simulink model "raspi_multicore_MPCtest_estDis"  (R2021b)
settings: Solver=FixedStepAuto  StartTime=0.0  StopTime=600  FixedStep=0.006  RelTol=1e-3  EnableMultiTasking=on
InitFcn:
  | %hardwareSetup;
values from neighbouring files (symbols this model uses):
  T_gait = 0.6    [MPCGen_OffsetFree.m]    (also in MPCGen_OffsetFree_UD.m = 0.65; MPCGen_OffsetFree_estDis.m; MPCcontrollerGen_OffsetFree.m = 0.7; MPCcontrollerGen_OffsetFree_UD.m = 0.65)
  Ts = 0.025    [MPCGen_OffsetFree.m]    (also in MPCGen_OffsetFree_UD.m = 0.02; MPCGen_OffsetFree_estDis.m = 0.03; MPCcontrollerGen_OffsetFree.m; MPCcontrollerGen_OffsetFree_UD.m = 0.02)
  Ts_DynSim = 0.005    [MPCGen_OffsetFree.m]    (also in MPCGen_OffsetFree_UD.m; MPCGen_OffsetFree_estDis.m = 0.006; MPCcontrollerGen_OffsetFree.m; MPCcontrollerGen_OffsetFree_UD.m)
libraries: PuppyLibrary x5, mpclib x1, slctrlblks x1
(part 2 of 2)

== matlab function raspi_multicore_MPCtest_estDis/MATLAB Function3 ==
  data: Xnow input; pCoM output; vCoM output; RPY output; Omega output
function [pCoM,vCoM,RPY,Omega] = fcn(Xnow)
pCoM=reshape(Xnow(1:3),3,1);
vCoM=reshape(Xnow(7:9),3,1);
RPY=reshape(Xnow(4:6),3,1);
Omega=reshape(Xnow(10:12),3,1);

== matlab function raspi_multicore_MPCtest_estDis/slopeGen1 ==
  data: slope input; sura output; startX input
function sura = fcn(slope,startX)
slope=slope/180*pi;
surP1=[startX;1;0];
surP2=[startX;-1;0];
surP3=[startX+1;0;tan(slope)];
W=[1,surP1(1:2)';
    1,surP2(1:2)';
    1,surP3(1:2)'];

sura=(W'*W)\W'*[surP1(3);surP2(3);surP3(3);];

== matlab function raspi_multicore_MPCtest_estDis/terrainSimulator1 ==
  data: surP1 input; touchInd output; surP2 input; xBP input; pendAll input; phi input; zSur output
function [touchInd,zSur] = fcn(surP1,surP2,xBP,pendAll,phi)
touchInd=zeros(4,1);
zSur=zeros(4,1);
LegState=[1;0;0;1];
s=phi/pi;
if phi>pi
    LegState=[0;1;1;0];
    s=s-1;
end
for i=1:1:4
    if LegState(i)<0.5 && s>0.2
        if pendAll(1,i)<xBP
            zSur(i)=[1;pendAll(1:2,i)]'*surP1;
        else
            zSur(i)=[1;pendAll(1:2,i)]'*surP2;
        end
        if pendAll(3,i)-zSur(i)<=0.001
            touchInd(i)=1;
        end
    end
end
end

== matlab function raspi_multicore_MPCtest_estDis/MATLAB Function4 ==
  data: SP input; zSur output size=[4,1]; SPLeg input; phi input; touchInd output size=[4,1]; OscStop input; LegState output size=[4,1]
function [zSur,touchInd,LegState] = fcn(SP,SPLeg,phi,OscStop)
zSur=reshape(SP(3,:),4,1);
LegState=[1;0;0;1];
touchInd=SPLeg;
s=phi/pi;
if phi>pi
    s=s-1;
    LegState=[0;1;1;0];
end
if abs(OscStop-1)<0.1
    LegState=[1;1;1;1];
end

for i=1:1:4
    if LegState(i)<0.5 && s>0.5
        if SPLeg(i)>0.5
            touchInd(i)=1;
        end
    end
end

== stateflow chart raspi_multicore_MPCtest_estDis/Chart ==
  state StandBy
    entry:
    estEN=0;
    oscEN=0;
    mpcSTOP=1;
  state step_enable
    entry:
    estEN=0;
    oscEN=1;
    mpcSTOP=0;
  state MPC_enable_p1
    entry:
    estEN=1;
    oscEN=0;
    mpcSTOP=1;
  state MPC_enable_p2
    entry:
    estEN=0;
    oscEN=0;
    mpcSTOP=0;
  state StandBy2
    entry:
    estEN=1;
    oscEN=0;
    mpcSTOP=1;
  state StandBy1
    entry:
    estEN=0;
    oscEN=0;
    mpcSTOP=1;
  (default) -> StandBy
  StandBy -> MPC_enable_p1 : [standEdge==1]
  MPC_enable_p1 -> MPC_enable_p2 : [after(1,sec)]
  MPC_enable_p2 -> step_enable : [stepEdge==1]
  StandBy2 -> StandBy : [after(1,sec)]
  step_enable -> StandBy1 : [stepEdge==1]
  StandBy1 -> StandBy2 : [after(1,sec)]
  data: estEN output size=[1,1]; oscEN output size=[1,1]; stepEdge input size=[1,1]; mpcSTOP output size=[1,1]; standEdge input size=[1,1]

== matlab function raspi_multicore_MPCtest_estDis/MATLAB Function6 ==
  data: u input; y output size=[13 1]
function y = index_array(u)
y = u(1,1:13)';

== matlab function raspi_multicore_MPCtest_estDis/MATLAB Function ==
  data: leftaxis input; vxPercent output size=[1,1]; rightaxis input; vyPercent output size=[1,1]; wzPercent output size=[1,1]; Left input; Right input
function [vxPercent,vyPercent,wzPercent] = fcn(leftaxis,rightaxis,Left,Right)
vxPercent=leftaxis(1);
vyPercent=-rightaxis(2);
%wzPercent=-rightaxis(2);
if Left>0.5
    wzPercent=1;
elseif Right>0.5
    wzPercent=-1;
else
    wzPercent=0;
end

== matlab function raspi_multicore_MPCtest_estDis/MATLAB Function7 ==
  data: u input; disable input; ori_xFB input; estDis output; estScale input; pCoM2 output; RPY2 output; vCoM2 output; omega2 output
function [estDis,pCoM2,RPY2,vCoM2,omega2] = fcn(u,disable,ori_xFB,estScale)
estDis = u(14:19)*estScale;
if disable<0.5
    pCoM2=u(1:3);
    RPY2=u(4:6);
    vCoM2=u(7:9);
    omega2=u(10:12);
else
    pCoM2=ori_xFB(1:3);
    RPY2=ori_xFB(4:6);
    vCoM2=ori_xFB(7:9);
    omega2=ori_xFB(10:12);
    estDis=0*estDis;
end

== matlab function raspi_multicore_MPCtest_estDis/MATLAB Function8 ==
  data: u input; uOut output size=[12 1]; DisFlag input
function uOut = fcn(u,DisFlag)
if DisFlag>0.5
    uOut=[0;0;7.5;0;0;7.5;0;0;7.5;0;0;7.5];
else
    uOut=u;
end

== matlab function raspi_multicore_MPCtest_estDis/Subsystem_Compound/MATLAB Function ==
  data: xhat input size=[21,1]; pCoM output size=[3,1]; vCoM output size=[3,1]; pArray_W output
function [pCoM,vCoM,pArray_W] = fcn(xhat)
% pB the CoM position in the world coordinate
% vB the CoM velocity
% Wpi the foot-end position in the world coordinate
pCoM=[xhat(1);xhat(2);xhat(3)];
vCoM=[xhat(4);xhat(5);xhat(6)];
pArray_W=xhat(7:18);

== matlab function raspi_multicore_MPCtest_estDis/Subsystem_Compound/MATLAB Function1 ==
  data: pArray_B input size=[12,1]; RPY input size=[3,1]; X0 output size=[21,1]; P0 output size=[21,21]; pArray_W0 output size=[12,1]
function [X0,P0,pArray_W0]=fcn(pArray_B,RPY)
% NOTE: pArray_W0 is calculated without the value of yaw angle!!!
Ry=[cos(RPY(2)),0,sin(RPY(2));
    0,1,0;
    -sin(RPY(2)),0,cos(RPY(2))];
Rx=[1,0,0;
    0,cos(RPY(1)),-sin(RPY(1));
    0,sin(RPY(1)),cos(RPY(1))];
pArray_B=reshape(pArray_B,3,4)/1000;
pArray_float=Ry*Rx*pArray_B; % foot-end position in floating coordinate
zOff=-min(pArray_float(3,:));
temp=pArray_float+[0;0;zOff]*[1,1,1,1];
pCoM=[0;0;zOff];
vCoM=[0;0;0];
pArray_W0=[temp(:,1);temp(:,2);temp(:,3);temp(:,4)];
X0=zeros(21,1);
X0(1:3)=pCoM;
X0(4:6)=vCoM;
X0(7:18)=reshape(pArray_W0,12,1);
X0(19:21)=zeros(3,1);
% X0=[pCoM;vCoM;reshape(pArray_W0,12,1);zeros(3,1)];
P0=eye(21)*1;

== stateflow chart raspi_multicore_MPCtest_estDis/JoyStick state machine ==
  state TurnRight
    entry:
    TurnLeft=0;
    TurnRight=1;
  state Stop
    entry:
    PhaseOscEN=0;
  state Flat2Slope
    entry:
    TransCommand=1;
  state Forward
    entry:
    PhaseOscEN=1;
    ForwardAmp=1;
    AngleOffset=0;
    TurnLeft=0;
    TurnRight=0;
  state StandBy
    entry:
    PhaseOscEN=0;
    ForwardAmp=0;
    AngleOffset=0;
    TurnLeft=0;
    TurnRight=0;
    TransCommand=0;
  state ClearAngle
    entry:
    AngleOffset=1;
  state OnSpot
    entry:
    PhaseOscEN=1;
    ForwardAmp=0;
    AngleOffset=0;
    TurnLeft=0;
    TurnRight=0;
  state Continue
    entry:
    PhaseOscEN=1;
  state TurnLeft
    entry:
    TurnLeft=1;
    TurnRight=0;
  OnSpot -> TurnRight [order 2] : [JS_number==0 && JS_value>1000]
  TurnRight -> OnSpot [order 2] : [JS_number==0 && JS_value>1000 && ForwardAmp==0 && after(0.1,sec)]
  Forward -> TurnRight [order 1] : [JS_number==0 && JS_value>1000]
  TurnRight -> Forward [order 1] : [JS_number==0 && JS_value>1000 && ForwardAmp==1 && after(0.1,sec)]
  (default) -> StandBy
  Flat2Slope -> Stop : [JS_number==3 && JS_value==1]
  OnSpot -> Forward [order 1] : [JS_number==1 && JS_value<-1000]
  Forward -> Flat2Slope [order 2] : [JS_number==4 && JS_value==1]
  ClearAngle -> OnSpot : [after(1,sec)]
  StandBy -> ClearAngle : [JS_number==3 && JS_value==1]
  TurnLeft -> Forward [order 1] : [JS_number==0 && JS_value<-1000 && ForwardAmp==1 && after(0.1,sec)]
  Forward -> OnSpot [order 4] : [JS_number==1 && JS_value<-1000]
  Forward -> TurnLeft [order 3] : [JS_number==0 && JS_value<-1000]
  Stop -> Continue : [JS_number==3 && JS_value==1 && after(0.1,sec)]
  Continue -> Stop : [JS_number==3 && JS_value==1 && after(0.1,sec)]
  OnSpot -> StandBy [order 3] : [JS_number==3 && JS_value==1]
  OnSpot -> TurnLeft [order 4] : [JS_number==0 && JS_value<-1000]
  TurnLeft -> OnSpot [order 2] : [JS_number==0 && JS_value<-1000 && ForwardAmp==0 && after(0.1,sec)]
  data: JS_number input; JS_value input; TurnRight output; AngleOffset output; PhaseOscEN output; TurnLeft output; ForwardAmp output; TransCommand output

== matlab function raspi_multicore_MPCtest_estDis/MATLAB Function1 ==
  data: u input; y output size=[13 1]
function y = index_array(u)
y = u(2,1:13)';

== matlab function raspi_multicore_MPCtest_estDis/MATLAB Function9 ==
  data: vx input; holdFlag output; vy input; EN input
function holdFlag = fcn(vx,vy,EN)

if abs(vx)<0.001 && abs(vy)<0.001
    holdFlag=0;
else
    holdFlag=1;
end
if EN<0.5
    holdFlag=0;
end

== matlab function raspi_multicore_MPCtest_estDis/online Constraints1 ==
  data: SPLeg input; E output size=[32 12]; F output size=[32 13]; G output size=[32 1]; surVN input; surV1 input; surV2 input; headG input; S output size=[32 6]
function [E,F,G,S] = fcn(SPLeg,surVN,surV1,surV2,headG)
% surVN: unit norm vector of the surface
% surV1: unit actangular vector 1 of the surface
% surV2: unit actangular vector 2 of the surface
% headG: robot heading vector in world coordinate

S=zeros(32,6);
%%%%%%%% set constraints %%%%%%%%%%
miu=0.4;
deltaFz=50; % w.r.t body coordinate
deltaFx=50; % w.r.t body coordinate
maxFz=70; % w.r.t. body coordinate
minFz=0;
maxRoll=10/180*pi;
minRoll=-10/180*pi;
maxPit=10/180*pi;
minPit=-10/180*pi;

% friction cone----------------------
Eb2=zeros(8,12);
Gb2=zeros(8,1);
%Vb2=ones(8,1);
for i=1:1:4
    Eb2(i,3*i-2:3*i)=-miu*surVN+surV1;
    Eb2(i+4,3*i-2:3*i)=-miu*surVN-surV1;
end
Eb3=zeros(8,12);
Gb3=zeros(8,1);
%Vb3=ones(8,1);
for i=1:1:4
    Eb3(i,3*i-2:3*i)=-miu*surVN+surV2;
    Eb3(i+4,3*i-2:3*i)=-miu*surVN-surV2;
end
% payload balance--------------
surVhead=headG-headG'*surVN*surVN;
surVhead=surVhead/norm(surVhead);
Eb4=zeros(4,12);
Gb4=zeros(4,1);
%Vb4=ones(4,1);
Eb4(1,1:3)=surVhead;
Eb4(1,10:12)=-surVhead;
Eb4(2,1:3)=-surVhead;
Eb4(2,10:12)=surVhead;
Gb4(1)=deltaFx;
Gb4(2)=deltaFx;
Eb4(3,4:6)=surVhead;
Eb4(3,7:9)=-surVhead;
Eb4(4,4:6)=-surVhead;
Eb4(4,7:9)=surVhead;
Gb4(3)=deltaFx;
Gb4(4)=deltaFx;

Eb5=zeros(4,12);
Gb5=zeros(4,1);
%Vb5=ones(4,1);
Eb5(1,1:3)=surVN;
Eb5(1,10:12)=-surVN;
Eb5(2,1:3)=-surVN;
Eb5(2,10:12)=surVN;
Gb5(1)=deltaFz;
Gb5(2)=deltaFz;
Eb5(3,4:6)=surVN;
Eb5(3,7:9)=-surVN;
Eb5(4,4:6)=-surVN;
Eb5(4,7:9)=surVN;
Gb5(3)=deltaFz;
Gb5(4)=deltaFz;

% support force greater than zero, gait define----------
Eb1=zeros(8,12);
Gb1=zeros(8,1);
Vb1=ones(8,1)*0.1;
for i=1:1:4
    Eb1(i,3*i-2:3*i)=surVN;
    Eb1(i+4,3*i-2:3*i)=-surVN;
    Gb1(i)=maxFz;
    Gb1(i+4)=-minFz;
end

for i=1:1:4
    if SPLeg(i)<0.5
        Gb1(i)=0;
        Gb1(i+4)=0;
    end
end

% restrictions for roll and pitch angle
% EA=zeros(4,12);
% GA=zeros(4,1);
% FA=zeros(4,13);
% FA(1,:)=[0,0,0,1,0,0,0,0,0,0,0,0,0];
% FA(2,:)=[0,0,0,-1,0,0,0,0,0,0,0,0,0];
% FA(3,:)=[0,0,0,0,1,0,0,0,0,0,0,0,0];
% FA(4,:)=[0,0,0,0,-1,0,0,0,0,0,0,0,0];
% GA(1)=maxPit;
% GA(2)=-minPit;
% GA(3)=maxRoll;
% GA(4)=-minRoll;



E=[Eb2;Eb3;Eb4;Eb5;Eb1];
F=[zeros(32,13)];
G=[Gb2;Gb3;Gb4;Gb5;Gb1];
%V=[Vb2;Vb3;Vb4;Vb5;Vb1];

% E=[Eb2;Eb3;Eb1];
% F=zeros(24,13);
% G=[Gb2;Gb3;Gb1];

%V=[Vb2;Vb3;Vb4;Vb5;Vb1];

== matlab function raspi_multicore_MPCtest_estDis/MATLAB Function5 ==
  data: u input; disable input; ori_xFB input; estDis output size=[6 1]; estScale input; pCoM2 output size=[3,1]; RPY2 output size=[3,1]; vCoM2 output size=[3,1]; omega2 output size=[3,1]
function [estDis,pCoM2,RPY2,vCoM2,omega2] = fcn(u,disable,ori_xFB,estScale)
estDis = u(14:19)*estScale;
if disable<0.5
    pCoM2=u(1:3);
    RPY2=u(4:6);
    vCoM2=u(7:9);
    omega2=u(10:12);
else
    pCoM2=ori_xFB(1:3);
    RPY2=ori_xFB(4:6);
    vCoM2=ori_xFB(7:9);
    omega2=ori_xFB(10:12);
    estDis=0*estDis;
end

== matlab function raspi_multicore_MPCtest_estDis/Subsystem/MATLAB Function ==
  data: xhat input size=[9,1]; pCoM output size=[3,1]; vCoM output size=[3,1]; pArray_B input; RPY input; pArray_W output
function [pCoM,vCoM,pArray_W] = fcn(xhat,pArray_B,RPY)
% pB the CoM position in the world coordinate
% vB the CoM velocity
% Wpi the foot-end position in the world coordinate
pCoM=[xhat(1);xhat(2);xhat(3)];
vCoM=[xhat(4);xhat(5);xhat(6)];
Rz=[cos(RPY(3)),-sin(RPY(3)),0;
    sin(RPY(3)),cos(RPY(3)),0;
    0,0,1];
Ry=[cos(RPY(2)),0,sin(RPY(2));
    0,1,0;
    -sin(RPY(2)),0,cos(RPY(2))];
Rx=[1,0,0;
    0,cos(RPY(1)),-sin(RPY(1));
    0,sin(RPY(1)),cos(RPY(1))];
R=Rz*Ry*Rx;
pArray_B=reshape(pArray_B,3,4)/1000;
temp=R*pArray_B+pCoM*[1,1,1,1];
pArray_W=[temp(:,1);temp(:,2);temp(:,3);temp(:,4)];
